simulink model "powertrain"  (R2019a)
settings: Solver=ode4  StartTime=0.0  StopTime=50  FixedStep=.01  RelTol=1e-3
undefined symbols (not defined in the file): Motor, quadModel
libraries: simulink x8
(part 2 of 2)

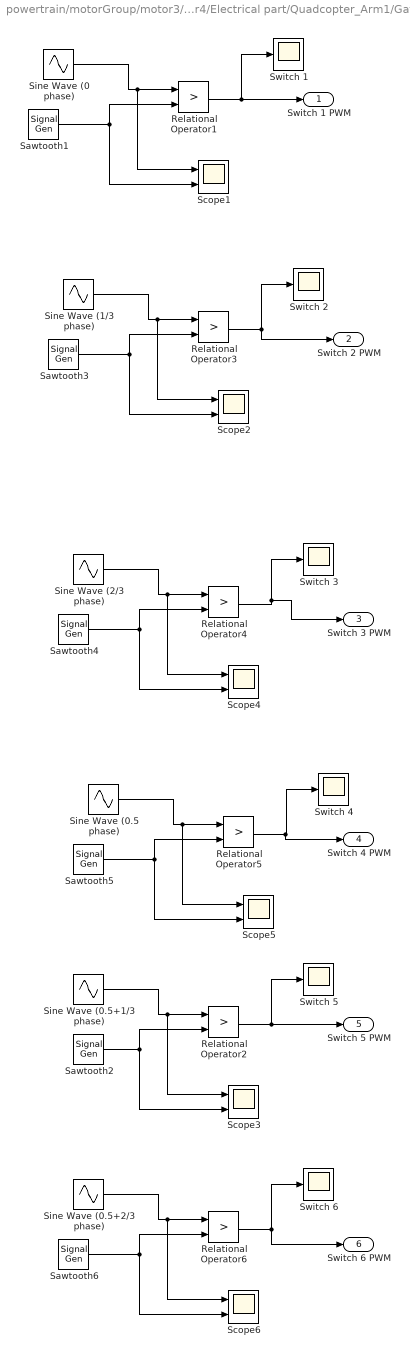
== system powertrain/motorGroup/motor3/motorRotor4/Electrical part/Quadcopter_Arm1/Gate Driver ==
  Relational Operator{1..6} (6 alike) : RelationalOperator  Operator=>  OutDataTypeStr=boolean  RndMeth=Simplest
  Sawtooth{1..6} (6 alike) : SignalGenerator  WaveForm=sawtooth  Frequency=20
  Scope{1..6} (6 alike) : Scope  NumInputPorts=2
  Sine Wave (0 phase) : Sin  Frequency=2*pi  SampleTime=0.001
  Sine Wave (0.5 phase) : Sin  Frequency=2*pi  Phase=0.5*(2*pi)  SampleTime=0.001
  Sine Wave (0.5+1/3 phase) : Sin  Frequency=2*pi  Phase=(0.5 + 1/3)*(2*pi)  SampleTime=0.001
  Sine Wave (0.5+2/3 phase) : Sin  Frequency=2*pi  Phase=(2/3 + 0.5)*2*pi  SampleTime=0.001
  Sine Wave (1/3 phase) : Sin  Frequency=2*pi  Phase=(1/3)*(2*pi)  SampleTime=0.001
  Sine Wave (2/3 phase) : Sin  Frequency=2*pi  Phase=(2/3)*(2*pi)  SampleTime=0.001
  Switch {1..6} (6 alike) : Scope
  Switch 1 PWM : Outport
  Switch 2 PWM : Outport  Port=2
  Switch 3 PWM : Outport  Port=3
  Switch 4 PWM : Outport  Port=4
  Switch 5 PWM : Outport  Port=5
  Switch 6 PWM : Outport  Port=6
  wires:
  Relational Operator4/1 -> Switch 3 PWM/1, Switch 3/1
  Sine Wave (1/3 phase)/1 -> Scope2/1, Relational Operator3/1
  Relational Operator6/1 -> Switch 6 PWM/1, Switch 6/1
  Sine Wave (2/3 phase)/1 -> Scope4/1, Relational Operator4/1
  Sawtooth4/1 -> Scope4/2, Relational Operator4/2
  Sawtooth1/1 -> Scope1/2, Relational Operator1/2
  Relational Operator2/1 -> Switch 5 PWM/1, Switch 5/1
  Sine Wave (0.5+2/3 phase)/1 -> Scope6/1, Relational Operator6/1
  Sawtooth5/1 -> Scope5/2, Relational Operator5/2
  Relational Operator1/1 -> Switch 1 PWM/1, Switch 1/1
  Sawtooth6/1 -> Scope6/2, Relational Operator6/2
  Sine Wave (0 phase)/1 -> Scope1/1, Relational Operator1/1
  Sine Wave (0.5 phase)/1 -> Scope5/1, Relational Operator5/1
  Relational Operator3/1 -> Switch 2 PWM/1, Switch 2/1
  Sine Wave (0.5+1/3 phase)/1 -> Scope3/1, Relational Operator2/1
  Sawtooth2/1 -> Scope3/2, Relational Operator2/2
  Sawtooth3/1 -> Scope2/2, Relational Operator3/2
  Relational Operator5/1 -> Switch 4 PWM/1, Switch 4/1

== system powertrain/motorGroup/motor4/motorRotor4/Electrical part/Quadcopter_Arm1/Delta Motor ==
  Vab : Inport
  Vbc : Inport  Port=2
  Vca : Inport  Port=3
  1/Lm : Gain  Gain=100
  1/Lm1 : Gain  Gain=100
  1/Lm2 : Gain  Gain=100
  Integrator : Integrator
  Integrator1 : Integrator
  Integrator2 : Integrator
  Mux : Mux  Inputs=1
  Rm : Gain  Gain=5
  Rm1 : Gain  Gain=5
  Rm2 : Gain  Gain=5
  motor current : Scope  NumInputPorts=3
  sum{,1..5} (6 alike) : Sum  Inputs=+-
  Out1 : Outport
  wires:
  1/Lm2/1 -> Integrator2/1
  Integrator/1 -> sum5/2, sum3/1, Rm/1
  sum3/1 -> Mux/1, motor current/1  "i1"
  Vab/1 -> sum/1
  Rm/1 -> sum/2
  Integrator1/1 -> sum4/1, sum3/2, Rm1/1
  sum1/1 -> 1/Lm1/1
  sum/1 -> 1/Lm/1
  1/Lm1/1 -> Integrator1/1
  Integrator2/1 -> sum5/1, sum4/2, Rm2/1
  1/Lm/1 -> Integrator/1
  sum4/1 -> motor current/2  "i2"
  Rm1/1 -> sum1/2
  Vca/1 -> sum2/1
  sum5/1 -> motor current/3  "i3"
  sum2/1 -> 1/Lm2/1
  Rm2/1 -> sum2/2
  Vbc/1 -> sum1/1
  Mux/1 -> Out1/1

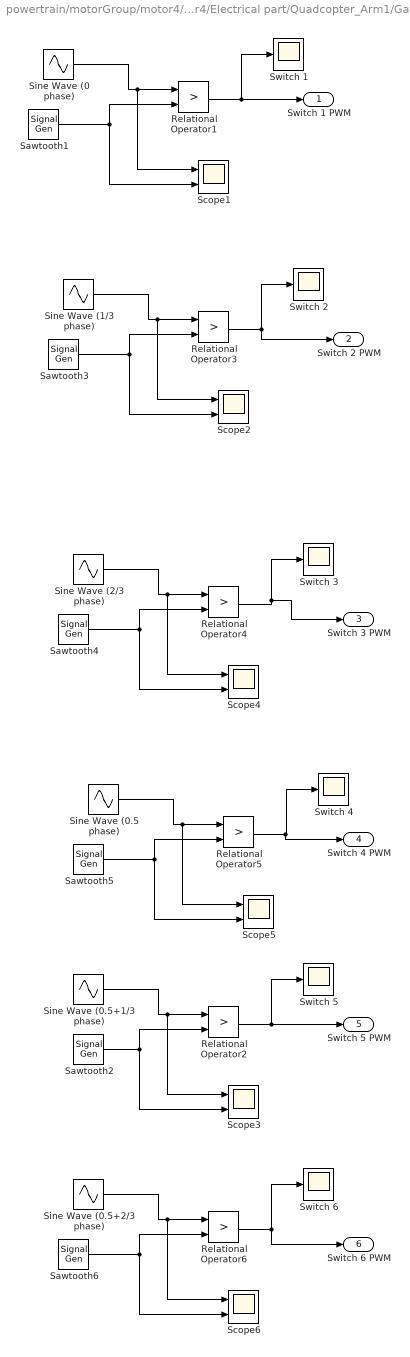
== system powertrain/motorGroup/motor4/motorRotor4/Electrical part/Quadcopter_Arm1/Gate Driver ==
  Relational Operator{1..6} (6 alike) : RelationalOperator  Operator=>  OutDataTypeStr=boolean  RndMeth=Simplest
  Sawtooth{1..6} (6 alike) : SignalGenerator  WaveForm=sawtooth  Frequency=20
  Scope{1..6} (6 alike) : Scope  NumInputPorts=2
  Sine Wave (0 phase) : Sin  Frequency=2*pi  SampleTime=0.001
  Sine Wave (0.5 phase) : Sin  Frequency=2*pi  Phase=0.5*(2*pi)  SampleTime=0.001
  Sine Wave (0.5+1/3 phase) : Sin  Frequency=2*pi  Phase=(0.5 + 1/3)*(2*pi)  SampleTime=0.001
  Sine Wave (0.5+2/3 phase) : Sin  Frequency=2*pi  Phase=(2/3 + 0.5)*2*pi  SampleTime=0.001
  Sine Wave (1/3 phase) : Sin  Frequency=2*pi  Phase=(1/3)*(2*pi)  SampleTime=0.001
  Sine Wave (2/3 phase) : Sin  Frequency=2*pi  Phase=(2/3)*(2*pi)  SampleTime=0.001
  Switch {1..6} (6 alike) : Scope
  Switch 1 PWM : Outport
  Switch 2 PWM : Outport  Port=2
  Switch 3 PWM : Outport  Port=3
  Switch 4 PWM : Outport  Port=4
  Switch 5 PWM : Outport  Port=5
  Switch 6 PWM : Outport  Port=6
  wires:
  Relational Operator4/1 -> Switch 3 PWM/1, Switch 3/1
  Sine Wave (1/3 phase)/1 -> Scope2/1, Relational Operator3/1
  Relational Operator6/1 -> Switch 6 PWM/1, Switch 6/1
  Sine Wave (2/3 phase)/1 -> Scope4/1, Relational Operator4/1
  Sawtooth4/1 -> Scope4/2, Relational Operator4/2
  Sawtooth1/1 -> Scope1/2, Relational Operator1/2
  Relational Operator2/1 -> Switch 5 PWM/1, Switch 5/1
  Sine Wave (0.5+2/3 phase)/1 -> Scope6/1, Relational Operator6/1
  Sawtooth5/1 -> Scope5/2, Relational Operator5/2
  Relational Operator1/1 -> Switch 1 PWM/1, Switch 1/1
  Sawtooth6/1 -> Scope6/2, Relational Operator6/2
  Sine Wave (0 phase)/1 -> Scope1/1, Relational Operator1/1
  Sine Wave (0.5 phase)/1 -> Scope5/1, Relational Operator5/1
  Relational Operator3/1 -> Switch 2 PWM/1, Switch 2/1
  Sine Wave (0.5+1/3 phase)/1 -> Scope3/1, Relational Operator2/1
  Sawtooth2/1 -> Scope3/2, Relational Operator2/2
  Sawtooth3/1 -> Scope2/2, Relational Operator3/2
  Relational Operator5/1 -> Switch 4 PWM/1, Switch 4/1

== matlab function powertrain/motorGroup/motor2/motorRotor4/Electrical part/Quadcopter_Arm1/Working MOSFET1 ==
  data: Vds input; Vgs input; R input; K input; Vth input; Vout output
function Vout   = MOSFET(Vds, Vgs, R, K, Vth)
Ids = 0;
Vd = 0;

    % if gate-source voltage does not exceed threshold, switch is open
    % no current through
    if Vgs <= Vth
        Vd = 0;
        Ids = 0;
        
    % if MOSFET is in linear region    
    elseif Vds<(Vgs-Vth)
        Vd = 20;
        Ids = K*(((Vgs - Vth)*Vds)-((Vds^2)/2));
        
     % if MOSFET is in saturation region   
    elseif (Vgs-Vth)<Vds
         Vd = 20;
         Ids = (K/2)*((Vgs-Vth)^2);         
    end

%calculate voltage output
%this voltage goes to the motor
Vout = Vd - Ids*R;

== matlab function powertrain/motorGroup/motor2/motorRotor4/Electrical part/Quadcopter_Arm1/Working MOSFET2 ==
  data: Vds input; Vgs input; R input; K input; Vth input; Vout output
function Vout   = MOSFET(Vds, Vgs, R, K, Vth)
Ids = 0;
Vd = 0;

    % if gate-source voltage does not exceed threshold, switch is open
    % no current through
    if Vgs <= Vth
        Vd = 0;
        Ids = 0;
        
    % if MOSFET is in linear region    
    elseif Vds<(Vgs-Vth)
        Vd = 20;
        Ids = K*(((Vgs - Vth)*Vds)-((Vds^2)/2));
        
     % if MOSFET is in saturation region   
    elseif (Vgs-Vth)<Vds
         Vd = 20;
         Ids = (K/2)*((Vgs-Vth)^2);         
    end

%calculate voltage output
%this voltage goes to the motor
Vout = Vd - Ids*R;

== matlab function powertrain/motorGroup/motor1/motorRotor4/Mechanical part/Propeller model  ==
  data: torque output; rpm input; thrust output
function [torque,thrust] = fcn(rpm)
% angular_velocity in rpm

%coefficient of thrust, empirically derived
coef_t = 2*(10^-15)*rpm^3 - 4*(10^-11)*rpm^2 + 3*(10^-7)*rpm + .1013;
%thrust = coef_t * density of air * velocity^2 * propeller diameter (m) ^4
thrust = coef_t*1.225*(rpm/60)^2*.2^4;
% empirically derived
torque = 4*(10^-14)*rpm^3 +  8*(10^-12)*rpm^2 + 3*(10^-6)*rpm;
end

== matlab function powertrain/motorGroup/motor2/motorRotor4/Electrical part/Quadcopter_Arm1/Working MOSFET3 ==
  data: Vds input; Vgs input; R input; K input; Vth input; Vout output
function Vout   = MOSFET(Vds, Vgs, R, K, Vth)
Ids = 0;
Vd = 0;

    % if gate-source voltage does not exceed threshold, switch is open
    % no current through
    if Vgs <= Vth
        Vd = 0;
        Ids = 0;
        
    % if MOSFET is in linear region    
    elseif Vds<(Vgs-Vth)
        Vd = 20;
        Ids = K*(((Vgs - Vth)*Vds)-((Vds^2)/2));
        
     % if MOSFET is in saturation region   
    elseif (Vgs-Vth)<Vds
         Vd = 20;
         Ids = (K/2)*((Vgs-Vth)^2);         
    end

%calculate voltage output
%this voltage goes to the motor
Vout = Vd - Ids*R;

== matlab function powertrain/motorGroup/motor2/motorRotor4/Electrical part/Quadcopter_Arm1/Working MOSFET4 ==
  data: Vds input; Vgs input; R input; K input; Vth input; Vout output
function Vout   = MOSFET(Vds, Vgs, R, K, Vth)
Ids = 0;
Vd = 0;

    % if gate-source voltage does not exceed threshold, switch is open
    % no current through
    if Vgs <= Vth
        Vd = 0;
        Ids = 0;
        
    % if MOSFET is in linear region    
    elseif Vds<(Vgs-Vth)
        Vd = 20;
        Ids = K*(((Vgs - Vth)*Vds)-((Vds^2)/2));
        
     % if MOSFET is in saturation region   
    elseif (Vgs-Vth)<Vds
         Vd = 20;
         Ids = (K/2)*((Vgs-Vth)^2);         
    end

%calculate voltage output
%this voltage goes to the motor
Vout = Vd - Ids*R;

== matlab function powertrain/motorGroup/motor2/motorRotor4/Electrical part/Quadcopter_Arm1/Working MOSFET5 ==
  data: Vds input; Vgs input; R input; K input; Vth input; Vout output
function Vout   = MOSFET(Vds, Vgs, R, K, Vth)
Ids = 0;
Vd = 0;

    % if gate-source voltage does not exceed threshold, switch is open
    % no current through
    if Vgs <= Vth
        Vd = 0;
        Ids = 0;
        
    % if MOSFET is in linear region    
    elseif Vds<(Vgs-Vth)
        Vd = 20;
        Ids = K*(((Vgs - Vth)*Vds)-((Vds^2)/2));
        
     % if MOSFET is in saturation region   
    elseif (Vgs-Vth)<Vds
         Vd = 20;
         Ids = (K/2)*((Vgs-Vth)^2);         
    end

%calculate voltage output
%this voltage goes to the motor
Vout = Vd - Ids*R;

== matlab function powertrain/motorGroup/motor2/motorRotor4/Electrical part/Quadcopter_Arm1/Working MOSFET6 ==
  data: Vds input; Vgs input; R input; K input; Vth input; Vout output
function Vout   = MOSFET(Vds, Vgs, R, K, Vth)
Ids = 0;
Vd = 0;

    % if gate-source voltage does not exceed threshold, switch is open
    % no current through
    if Vgs <= Vth
        Vd = 0;
        Ids = 0;
        
    % if MOSFET is in linear region    
    elseif Vds<(Vgs-Vth)
        Vd = 20;
        Ids = K*(((Vgs - Vth)*Vds)-((Vds^2)/2));
        
     % if MOSFET is in saturation region   
    elseif (Vgs-Vth)<Vds
         Vd = 20;
         Ids = (K/2)*((Vgs-Vth)^2);         
    end

%calculate voltage output
%this voltage goes to the motor
Vout = Vd - Ids*R;

== matlab function powertrain/motorGroup/motor2/motorRotor4/Mechanical part/Propeller model  ==
  data: torque output; rpm input; thrust output
function [torque,thrust] = fcn(rpm)
% angular_velocity in rpm

%coefficient of thrust, empirically derived
coef_t = 2*(10^-15)*rpm^3 - 4*(10^-11)*rpm^2 + 3*(10^-7)*rpm + .1013;
%thrust = coef_t * density of air * velocity^2 * propeller diameter (m) ^4
thrust = coef_t*1.225*(rpm/60)^2*.2^4;
% empirically derived
torque = 4*(10^-14)*rpm^3 +  8*(10^-12)*rpm^2 + 3*(10^-6)*rpm;
end

== matlab function powertrain/motorGroup/motor3/motorRotor4/Electrical part/Quadcopter_Arm1/Working MOSFET1 ==
  data: Vds input; Vgs input; R input; K input; Vth input; Vout output
function Vout   = MOSFET(Vds, Vgs, R, K, Vth)
Ids = 0;
Vd = 0;

    % if gate-source voltage does not exceed threshold, switch is open
    % no current through
    if Vgs <= Vth
        Vd = 0;
        Ids = 0;
        
    % if MOSFET is in linear region    
    elseif Vds<(Vgs-Vth)
        Vd = 20;
        Ids = K*(((Vgs - Vth)*Vds)-((Vds^2)/2));
        
     % if MOSFET is in saturation region   
    elseif (Vgs-Vth)<Vds
         Vd = 20;
         Ids = (K/2)*((Vgs-Vth)^2);         
    end

%calculate voltage output
%this voltage goes to the motor
Vout = Vd - Ids*R;

== matlab function powertrain/motorGroup/motor3/motorRotor4/Electrical part/Quadcopter_Arm1/Working MOSFET2 ==
  data: Vds input; Vgs input; R input; K input; Vth input; Vout output
function Vout   = MOSFET(Vds, Vgs, R, K, Vth)
Ids = 0;
Vd = 0;

    % if gate-source voltage does not exceed threshold, switch is open
    % no current through
    if Vgs <= Vth
        Vd = 0;
        Ids = 0;
        
    % if MOSFET is in linear region    
    elseif Vds<(Vgs-Vth)
        Vd = 20;
        Ids = K*(((Vgs - Vth)*Vds)-((Vds^2)/2));
        
     % if MOSFET is in saturation region   
    elseif (Vgs-Vth)<Vds
         Vd = 20;
         Ids = (K/2)*((Vgs-Vth)^2);         
    end

%calculate voltage output
%this voltage goes to the motor
Vout = Vd - Ids*R;

== matlab function powertrain/motorGroup/motor3/motorRotor4/Electrical part/Quadcopter_Arm1/Working MOSFET3 ==
  data: Vds input; Vgs input; R input; K input; Vth input; Vout output
function Vout   = MOSFET(Vds, Vgs, R, K, Vth)
Ids = 0;
Vd = 0;

    % if gate-source voltage does not exceed threshold, switch is open
    % no current through
    if Vgs <= Vth
        Vd = 0;
        Ids = 0;
        
    % if MOSFET is in linear region    
    elseif Vds<(Vgs-Vth)
        Vd = 20;
        Ids = K*(((Vgs - Vth)*Vds)-((Vds^2)/2));
        
     % if MOSFET is in saturation region   
    elseif (Vgs-Vth)<Vds
         Vd = 20;
         Ids = (K/2)*((Vgs-Vth)^2);         
    end

%calculate voltage output
%this voltage goes to the motor
Vout = Vd - Ids*R;

== matlab function powertrain/motorGroup/motor3/motorRotor4/Electrical part/Quadcopter_Arm1/Working MOSFET4 ==
  data: Vds input; Vgs input; R input; K input; Vth input; Vout output
function Vout   = MOSFET(Vds, Vgs, R, K, Vth)
Ids = 0;
Vd = 0;

    % if gate-source voltage does not exceed threshold, switch is open
    % no current through
    if Vgs <= Vth
        Vd = 0;
        Ids = 0;
        
    % if MOSFET is in linear region    
    elseif Vds<(Vgs-Vth)
        Vd = 20;
        Ids = K*(((Vgs - Vth)*Vds)-((Vds^2)/2));
        
     % if MOSFET is in saturation region   
    elseif (Vgs-Vth)<Vds
         Vd = 20;
         Ids = (K/2)*((Vgs-Vth)^2);         
    end

%calculate voltage output
%this voltage goes to the motor
Vout = Vd - Ids*R;

== matlab function powertrain/motorGroup/motor3/motorRotor4/Electrical part/Quadcopter_Arm1/Working MOSFET5 ==
  data: Vds input; Vgs input; R input; K input; Vth input; Vout output
function Vout   = MOSFET(Vds, Vgs, R, K, Vth)
Ids = 0;
Vd = 0;

    % if gate-source voltage does not exceed threshold, switch is open
    % no current through
    if Vgs <= Vth
        Vd = 0;
        Ids = 0;
        
    % if MOSFET is in linear region    
    elseif Vds<(Vgs-Vth)
        Vd = 20;
        Ids = K*(((Vgs - Vth)*Vds)-((Vds^2)/2));
        
     % if MOSFET is in saturation region   
    elseif (Vgs-Vth)<Vds
         Vd = 20;
         Ids = (K/2)*((Vgs-Vth)^2);         
    end

%calculate voltage output
%this voltage goes to the motor
Vout = Vd - Ids*R;

== matlab function powertrain/motorGroup/motor3/motorRotor4/Electrical part/Quadcopter_Arm1/Working MOSFET6 ==
  data: Vds input; Vgs input; R input; K input; Vth input; Vout output
function Vout   = MOSFET(Vds, Vgs, R, K, Vth)
Ids = 0;
Vd = 0;

    % if gate-source voltage does not exceed threshold, switch is open
    % no current through
    if Vgs <= Vth
        Vd = 0;
        Ids = 0;
        
    % if MOSFET is in linear region    
    elseif Vds<(Vgs-Vth)
        Vd = 20;
        Ids = K*(((Vgs - Vth)*Vds)-((Vds^2)/2));
        
     % if MOSFET is in saturation region   
    elseif (Vgs-Vth)<Vds
         Vd = 20;
         Ids = (K/2)*((Vgs-Vth)^2);         
    end

%calculate voltage output
%this voltage goes to the motor
Vout = Vd - Ids*R;

== matlab function powertrain/motorGroup/motor3/motorRotor4/Mechanical part/Propeller model  ==
  data: torque output; rpm input; thrust output
function [torque,thrust] = fcn(rpm)
% angular_velocity in rpm

%coefficient of thrust, empirically derived
coef_t = 2*(10^-15)*rpm^3 - 4*(10^-11)*rpm^2 + 3*(10^-7)*rpm + .1013;
%thrust = coef_t * density of air * velocity^2 * propeller diameter (m) ^4
thrust = coef_t*1.225*(rpm/60)^2*.2^4;
% empirically derived
torque = 4*(10^-14)*rpm^3 +  8*(10^-12)*rpm^2 + 3*(10^-6)*rpm;
end

== matlab function powertrain/motorGroup/motor4/motorRotor4/Electrical part/Quadcopter_Arm1/Working MOSFET1 ==
  data: Vds input; Vgs input; R input; K input; Vth input; Vout output
function Vout   = MOSFET(Vds, Vgs, R, K, Vth)
Ids = 0;
Vd = 0;

    % if gate-source voltage does not exceed threshold, switch is open
    % no current through
    if Vgs <= Vth
        Vd = 0;
        Ids = 0;
        
    % if MOSFET is in linear region    
    elseif Vds<(Vgs-Vth)
        Vd = 20;
        Ids = K*(((Vgs - Vth)*Vds)-((Vds^2)/2));
        
     % if MOSFET is in saturation region   
    elseif (Vgs-Vth)<Vds
         Vd = 20;
         Ids = (K/2)*((Vgs-Vth)^2);         
    end

%calculate voltage output
%this voltage goes to the motor
Vout = Vd - Ids*R;

== matlab function powertrain/motorGroup/motor4/motorRotor4/Electrical part/Quadcopter_Arm1/Working MOSFET2 ==
  data: Vds input; Vgs input; R input; K input; Vth input; Vout output
function Vout   = MOSFET(Vds, Vgs, R, K, Vth)
Ids = 0;
Vd = 0;

    % if gate-source voltage does not exceed threshold, switch is open
    % no current through
    if Vgs <= Vth
        Vd = 0;
        Ids = 0;
        
    % if MOSFET is in linear region    
    elseif Vds<(Vgs-Vth)
        Vd = 20;
        Ids = K*(((Vgs - Vth)*Vds)-((Vds^2)/2));
        
     % if MOSFET is in saturation region   
    elseif (Vgs-Vth)<Vds
         Vd = 20;
         Ids = (K/2)*((Vgs-Vth)^2);         
    end

%calculate voltage output
%this voltage goes to the motor
Vout = Vd - Ids*R;

== matlab function powertrain/motorGroup/motor1/motorRotor4/Electrical part/Quadcopter_Arm1/Working MOSFET1 ==
  data: Vds input; Vgs input; R input; K input; Vth input; Vout output
function Vout   = MOSFET(Vds, Vgs, R, K, Vth)
Ids = 0;
Vd = 0;

    % if gate-source voltage does not exceed threshold, switch is open
    % no current through
    if Vgs <= Vth
        Vd = 0;
        Ids = 0;
        
    % if MOSFET is in linear region    
    elseif Vds<(Vgs-Vth)
        Vd = 20;
        Ids = K*(((Vgs - Vth)*Vds)-((Vds^2)/2));
        
     % if MOSFET is in saturation region   
    elseif (Vgs-Vth)<Vds
         Vd = 20;
         Ids = (K/2)*((Vgs-Vth)^2);         
    end

%calculate voltage output
%this voltage goes to the motor
Vout = Vd - Ids*R;

== matlab function powertrain/motorGroup/motor1/motorRotor4/Electrical part/Quadcopter_Arm1/Working MOSFET2 ==
  data: Vds input; Vgs input; R input; K input; Vth input; Vout output
function Vout   = MOSFET(Vds, Vgs, R, K, Vth)
Ids = 0;
Vd = 0;

    % if gate-source voltage does not exceed threshold, switch is open
    % no current through
    if Vgs <= Vth
        Vd = 0;
        Ids = 0;
        
    % if MOSFET is in linear region    
    elseif Vds<(Vgs-Vth)
        Vd = 20;
        Ids = K*(((Vgs - Vth)*Vds)-((Vds^2)/2));
        
     % if MOSFET is in saturation region   
    elseif (Vgs-Vth)<Vds
         Vd = 20;
         Ids = (K/2)*((Vgs-Vth)^2);         
    end

%calculate voltage output
%this voltage goes to the motor
Vout = Vd - Ids*R;

== matlab function powertrain/motorGroup/motor1/motorRotor4/Electrical part/Quadcopter_Arm1/Working MOSFET3 ==
  data: Vds input; Vgs input; R input; K input; Vth input; Vout output
function Vout   = MOSFET(Vds, Vgs, R, K, Vth)
Ids = 0;
Vd = 0;

    % if gate-source voltage does not exceed threshold, switch is open
    % no current through
    if Vgs <= Vth
        Vd = 0;
        Ids = 0;
        
    % if MOSFET is in linear region    
    elseif Vds<(Vgs-Vth)
        Vd = 20;
        Ids = K*(((Vgs - Vth)*Vds)-((Vds^2)/2));
        
     % if MOSFET is in saturation region   
    elseif (Vgs-Vth)<Vds
         Vd = 20;
         Ids = (K/2)*((Vgs-Vth)^2);         
    end

%calculate voltage output
%this voltage goes to the motor
Vout = Vd - Ids*R;

== matlab function powertrain/motorGroup/motor1/motorRotor4/Electrical part/Quadcopter_Arm1/Working MOSFET4 ==
  data: Vds input; Vgs input; R input; K input; Vth input; Vout output
function Vout   = MOSFET(Vds, Vgs, R, K, Vth)
Ids = 0;
Vd = 0;

    % if gate-source voltage does not exceed threshold, switch is open
    % no current through
    if Vgs <= Vth
        Vd = 0;
        Ids = 0;
        
    % if MOSFET is in linear region    
    elseif Vds<(Vgs-Vth)
        Vd = 20;
        Ids = K*(((Vgs - Vth)*Vds)-((Vds^2)/2));
        
     % if MOSFET is in saturation region   
    elseif (Vgs-Vth)<Vds
         Vd = 20;
         Ids = (K/2)*((Vgs-Vth)^2);         
    end

%calculate voltage output
%this voltage goes to the motor
Vout = Vd - Ids*R;

== matlab function powertrain/motorGroup/motor1/motorRotor4/Electrical part/Quadcopter_Arm1/Working MOSFET5 ==
  data: Vds input; Vgs input; R input; K input; Vth input; Vout output
function Vout   = MOSFET(Vds, Vgs, R, K, Vth)
Ids = 0;
Vd = 0;

    % if gate-source voltage does not exceed threshold, switch is open
    % no current through
    if Vgs <= Vth
        Vd = 0;
        Ids = 0;
        
    % if MOSFET is in linear region    
    elseif Vds<(Vgs-Vth)
        Vd = 20;
        Ids = K*(((Vgs - Vth)*Vds)-((Vds^2)/2));
        
     % if MOSFET is in saturation region   
    elseif (Vgs-Vth)<Vds
         Vd = 20;
         Ids = (K/2)*((Vgs-Vth)^2);         
    end

%calculate voltage output
%this voltage goes to the motor
Vout = Vd - Ids*R;

== matlab function powertrain/motorGroup/motor1/motorRotor4/Electrical part/Quadcopter_Arm1/Working MOSFET6 ==
  data: Vds input; Vgs input; R input; K input; Vth input; Vout output
function Vout   = MOSFET(Vds, Vgs, R, K, Vth)
Ids = 0;
Vd = 0;

    % if gate-source voltage does not exceed threshold, switch is open
    % no current through
    if Vgs <= Vth
        Vd = 0;
        Ids = 0;
        
    % if MOSFET is in linear region    
    elseif Vds<(Vgs-Vth)
        Vd = 20;
        Ids = K*(((Vgs - Vth)*Vds)-((Vds^2)/2));
        
     % if MOSFET is in saturation region   
    elseif (Vgs-Vth)<Vds
         Vd = 20;
         Ids = (K/2)*((Vgs-Vth)^2);         
    end

%calculate voltage output
%this voltage goes to the motor
Vout = Vd - Ids*R;

== matlab function powertrain/motorGroup/motor4/motorRotor4/Electrical part/Quadcopter_Arm1/Working MOSFET3 ==
  data: Vds input; Vgs input; R input; K input; Vth input; Vout output
function Vout   = MOSFET(Vds, Vgs, R, K, Vth)
Ids = 0;
Vd = 0;

    % if gate-source voltage does not exceed threshold, switch is open
    % no current through
    if Vgs <= Vth
        Vd = 0;
        Ids = 0;
        
    % if MOSFET is in linear region    
    elseif Vds<(Vgs-Vth)
        Vd = 20;
        Ids = K*(((Vgs - Vth)*Vds)-((Vds^2)/2));
        
     % if MOSFET is in saturation region   
    elseif (Vgs-Vth)<Vds
         Vd = 20;
         Ids = (K/2)*((Vgs-Vth)^2);         
    end

%calculate voltage output
%this voltage goes to the motor
Vout = Vd - Ids*R;

== matlab function powertrain/motorGroup/motor4/motorRotor4/Electrical part/Quadcopter_Arm1/Working MOSFET4 ==
  data: Vds input; Vgs input; R input; K input; Vth input; Vout output
function Vout   = MOSFET(Vds, Vgs, R, K, Vth)
Ids = 0;
Vd = 0;

    % if gate-source voltage does not exceed threshold, switch is open
    % no current through
    if Vgs <= Vth
        Vd = 0;
        Ids = 0;
        
    % if MOSFET is in linear region    
    elseif Vds<(Vgs-Vth)
        Vd = 20;
        Ids = K*(((Vgs - Vth)*Vds)-((Vds^2)/2));
        
     % if MOSFET is in saturation region   
    elseif (Vgs-Vth)<Vds
         Vd = 20;
         Ids = (K/2)*((Vgs-Vth)^2);         
    end

%calculate voltage output
%this voltage goes to the motor
Vout = Vd - Ids*R;

== matlab function powertrain/motorGroup/motor4/motorRotor4/Electrical part/Quadcopter_Arm1/Working MOSFET5 ==
  data: Vds input; Vgs input; R input; K input; Vth input; Vout output
function Vout   = MOSFET(Vds, Vgs, R, K, Vth)
Ids = 0;
Vd = 0;

    % if gate-source voltage does not exceed threshold, switch is open
    % no current through
    if Vgs <= Vth
        Vd = 0;
        Ids = 0;
        
    % if MOSFET is in linear region    
    elseif Vds<(Vgs-Vth)
        Vd = 20;
        Ids = K*(((Vgs - Vth)*Vds)-((Vds^2)/2));
        
     % if MOSFET is in saturation region   
    elseif (Vgs-Vth)<Vds
         Vd = 20;
         Ids = (K/2)*((Vgs-Vth)^2);         
    end

%calculate voltage output
%this voltage goes to the motor
Vout = Vd - Ids*R;

== matlab function powertrain/motorGroup/motor4/motorRotor4/Electrical part/Quadcopter_Arm1/Working MOSFET6 ==
  data: Vds input; Vgs input; R input; K input; Vth input; Vout output
function Vout   = MOSFET(Vds, Vgs, R, K, Vth)
Ids = 0;
Vd = 0;

    % if gate-source voltage does not exceed threshold, switch is open
    % no current through
    if Vgs <= Vth
        Vd = 0;
        Ids = 0;
        
    % if MOSFET is in linear region    
    elseif Vds<(Vgs-Vth)
        Vd = 20;
        Ids = K*(((Vgs - Vth)*Vds)-((Vds^2)/2));
        
     % if MOSFET is in saturation region   
    elseif (Vgs-Vth)<Vds
         Vd = 20;
         Ids = (K/2)*((Vgs-Vth)^2);         
    end

%calculate voltage output
%this voltage goes to the motor
Vout = Vd - Ids*R;

== matlab function powertrain/motorGroup/motor4/motorRotor4/Mechanical part/Propeller model  ==
  data: torque output; rpm input; thrust output
function [torque,thrust] = fcn(rpm)
% angular_velocity in rpm

%coefficient of thrust, empirically derived
coef_t = 2*(10^-15)*rpm^3 - 4*(10^-11)*rpm^2 + 3*(10^-7)*rpm + .1013;
%thrust = coef_t * density of air * velocity^2 * propeller diameter (m) ^4
thrust = coef_t*1.225*(rpm/60)^2*.2^4;
% empirically derived
torque = 4*(10^-14)*rpm^3 +  8*(10^-12)*rpm^2 + 3*(10^-6)*rpm;
end
